simulink model "prova_P2_posicao"  (R2020a)
settings: Solver=VariableStepAuto  StartTime=0.0  StopTime=100.0  RelTol=1e-3
values from neighbouring files (symbols this model uses):
  Tz = 0.001    [ResultadosEnunciado.mat]
settings Model: Creator=jguil  LastModifiedBy=jguil

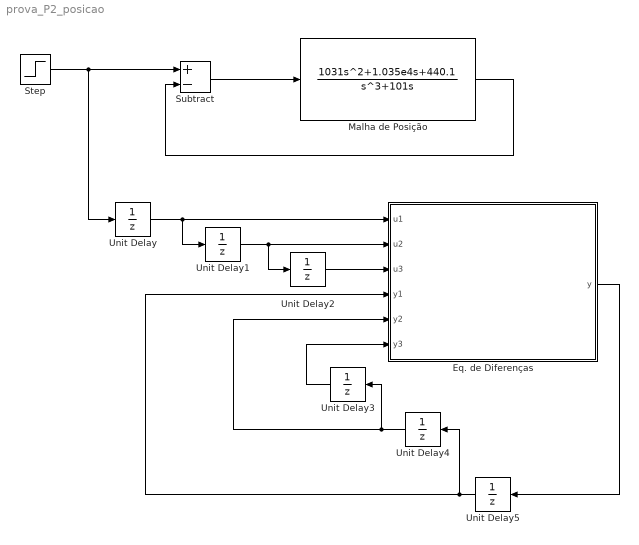
== system prova_P2_posicao ==
  Eq. de Diferenças : MATLAB Function  TreatAsAtomicUnit=on
  Malha de Posição : TransferFcn  Numerator=[1031 1.035e4 440.1]  Denominator=[1 0 101 0]
  Step : Step  SampleTime=0
  Subtract : Sum  Inputs=+-
  Unit Delay{,1..5} (6 alike) : UnitDelay  SampleTime=Tz  HasFrameUpgradeWarning=on
  wires:
  Malha de Posição/1 -> Subtract/2
  Step/1 -> Unit Delay/1, Subtract/1
  Subtract/1 -> Malha de Posição/1
  Unit Delay1/1 -> Unit Delay2/1, Eq. de Diferenças/2(u2)
  Unit Delay/1 -> Unit Delay1/1, Eq. de Diferenças/1(u1)
  Unit Delay2/1 -> Eq. de Diferenças/3(u3)
  Eq. de Diferenças/1(y) -> Unit Delay5/1
  Unit Delay5/1 -> Unit Delay4/1, Eq. de Diferenças/4(y1)
  Unit Delay4/1 -> Unit Delay3/1, Eq. de Diferenças/5(y2)
  Unit Delay3/1 -> Eq. de Diferenças/6(y3)

== matlab function prova_P2_posicao/Eq. de Diferenças ==
  data: u1 input; y output; u2 input; u3 input; y1 input; y2 input; y3 input
function y = aprox(u1,u2,u3,y1,y2,y3)

y = 1.96889135*y1-0.9482377876*y2-0.02065400366*y3+1.0310076497*u1-2.05166121*u2+1.020654004*u3;
